simulink model "fit_test"  (R2021a)
settings: Solver=VariableStepAuto  StartTime=0.0  StopTime=60.0  RelTol=1e-3
values from neighbouring files (symbols this model uses):
  beta = 0.6    [FES_setup.m]
  fit_min = 0    [FES_setup.m]
  freq = 30    [FES_setup.m]
  Tfat = 18    [FES_setup.m]
  Trec = 30    [FES_setup.m]
settings Model: Creator=nathanielgoldfarb  LastModifiedBy=nathanielgoldfarb

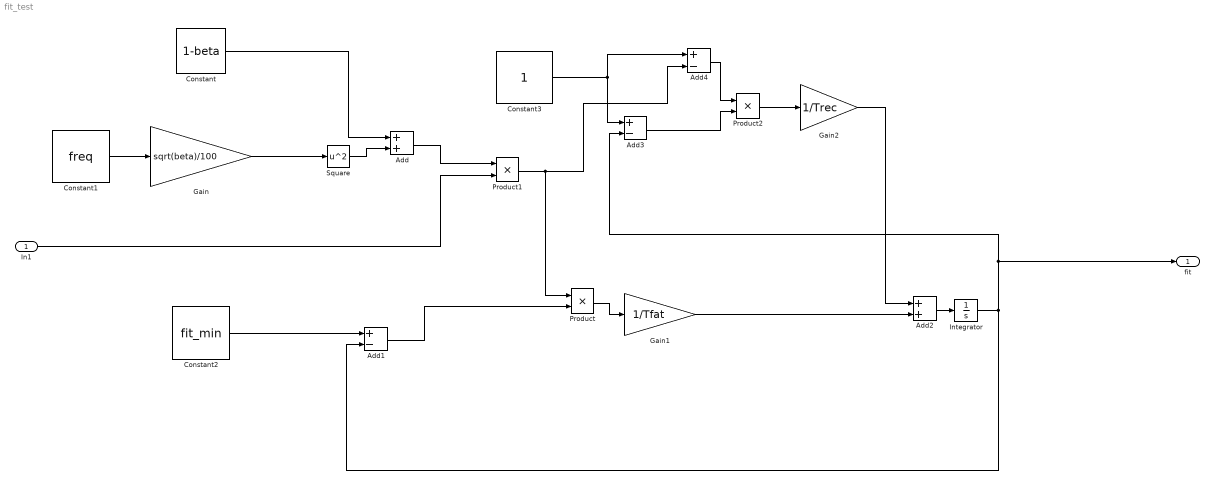
== system fit_test ==
  In1 : Inport
  Add : Sum
  Add1 : Sum  Inputs=+-
  Add2 : Sum
  Add3 : Sum  Inputs=+-
  Add4 : Sum  Inputs=+-
  Constant : Constant  Value=1-beta
  Constant1 : Constant  Value=freq
  Constant2 : Constant  Value=fit_min
  Constant3 : Constant
  Gain : Gain  Gain=sqrt(beta)/100
  Gain1 : Gain  Gain=1/Tfat
  Gain2 : Gain  Gain=1/Trec
  Integrator : Integrator  InitialCondition=1
  Product : Product
  Product1 : Product
  Product2 : Product
  Square : Math  Operator=square  SaturateOnIntegerOverflow=on
  fit : Outport
  wires:
  Constant1/1 -> Gain/1
  Gain/1 -> Square/1
  Square/1 -> Add/2
  Constant/1 -> Add/1
  Constant2/1 -> Add1/1
  Add2/1 -> Integrator/1
  Integrator/1 -> Add1/2, fit/1, Add3/2
  Product/1 -> Gain1/1
  Gain1/1 -> Add2/2
  Constant3/1 -> Add3/1, Add4/1
  Add/1 -> Product1/1
  Product1/1 -> Product/1, Add4/2
  Add1/1 -> Product/2
  Add4/1 -> Product2/1
  Add3/1 -> Product2/2
  Product2/1 -> Gain2/1
  Gain2/1 -> Add2/1
  In1/1 -> Product1/2
